simulink model "aufg2_schaltbild1"  (R2015a)
settings: Solver=ode45  StartTime=0.0  StopTime=10.0  RelTol=1e-3
settings Model: Creator=Daniel  LastModifiedBy=Daniel

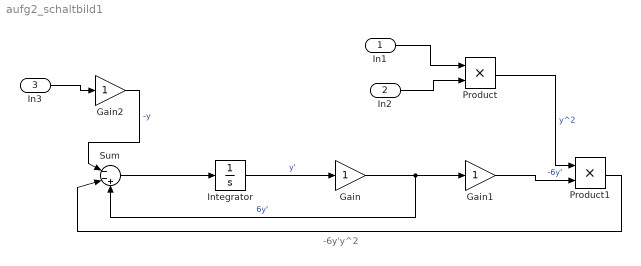
== system aufg2_schaltbild1 ==
  note: -6y'y^2
  In1 : Inport
  In2 : Inport  Port=2
  In3 : Inport  Port=3
  Gain : Gain
  Gain1 : Gain
  Gain2 : Gain
  Integrator : Integrator
  Product : Product
  Product1 : Product
  Sum : Sum  Inputs=|--+
  wires:
  In3/1 -> Gain2/1
  In1/1 -> Product/1
  In2/1 -> Product/2
  Integrator/1 -> Gain/1  "y'"
  Gain/1 -> Gain1/1, Sum/3  "6y'"
  Gain1/1 -> Product1/2  "-6y'"
  Product/1 -> Product1/1  "y^2"
  Product1/1 -> Sum/2
  Sum/1 -> Integrator/1
  Gain2/1 -> Sum/1  "-y"
